simulink model "classifyRealtimeSignals"  (R2019a)
settings: Solver=VariableStepAuto  StartTime=0.0  StopTime=inf  RelTol=1e-3
undefined symbols (not defined in the file or in its folder): daq
libraries: dspfdesign x3, dspxfrm3 x3, dspnetwork x2, daqlib x1
settings Model: Creator=Kusunoki  LastModifiedBy=Owner

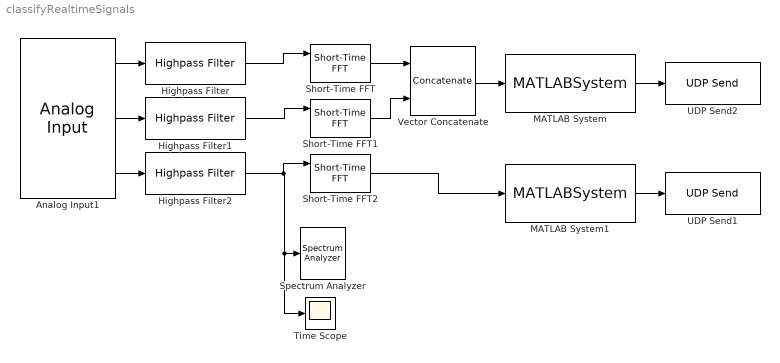
== system classifyRealtimeSignals ==
  Analog Input1 : daqlib/Analog Input  DeviceMenu=ni Dev1 (USB-6000)  Device=ni Dev1 (USB-6000)  ObjConstructor=daq.createSession('ni')  NChannelsSelected=3  Channels=1$ai0$$Dev1$1$1$1$1$#1$ai1$$Dev1$1$1$1$1$#1$ai2$$Dev1$1$1$1$1$#0$ai3$$Dev1$1$1$1$1$#0$ai4$$Dev1$1$1$1$1$#0$ai5$$Dev1$1$1$1$1$#0$ai6$$Dev1$1$1$1$1$#0$ai7$$Dev1$1$1$1$1$#  NPorts=1 per channel  SampleRate=2000  ActualRate=2000.5001  ScansPerTrigger=200  OutputTimestamp=off  AcqMode=0  NumFrameBuffer=100  OutputTriggertime=off
      settings: SourceProductName=Data Acquisition Toolbox  SourceProductBaseCode=DA
  Highpass Filter : dspfdesign/Highpass Filter  FilterType=FIR  DesignForMinimumOrder=on  FilterOrder=50  StopbandFrequency=8e3  PassbandFrequency=12e3  StopbandAttenuation=80  PassbandRipple=0.1  InheritSampleRate=off  SampleRate=44100  SimulateUsing=Interpreted execution  roundingMode=Floor  coeffsDataTypeStr=fixdt(1,16)
      settings: SourceProductName=DSP System Toolbox
  Highpass Filter1 : dspfdesign/Highpass Filter  FilterType=FIR  DesignForMinimumOrder=on  FilterOrder=50  StopbandFrequency=8e3  PassbandFrequency=12e3  StopbandAttenuation=80  PassbandRipple=0.1  InheritSampleRate=off  SampleRate=44100  SimulateUsing=Interpreted execution  roundingMode=Floor  coeffsDataTypeStr=fixdt(1,16)
      settings: SourceProductName=DSP System Toolbox
  Highpass Filter2 : dspfdesign/Highpass Filter  FilterType=FIR  DesignForMinimumOrder=on  FilterOrder=50  StopbandFrequency=8e3  PassbandFrequency=12e3  StopbandAttenuation=80  PassbandRipple=0.1  InheritSampleRate=off  SampleRate=44100  SimulateUsing=Interpreted execution  roundingMode=Floor  coeffsDataTypeStr=fixdt(1,16)
      settings: SourceProductName=DSP System Toolbox
  MATLAB System : MATLABSystem  System=NetEEG  net=[]  SimulateUsing=Code generation
      mask Type: NetEEG
      mask Display:
      | disp('NetEEG');
      | port_label('input',1,'u');
      | port_label('output',1,'y');
  MATLAB System1 : MATLABSystem  System=NetEMG  net=[]  SimulateUsing=Code generation
      mask Type: NetEMG
      mask Display:
      | disp('NetEMG');
      | port_label('input',1,'u');
      | port_label('output',1,'y');
  Short-Time FFT : dspxfrm3/Short-Time FFT  W=512  OvLap=384  M=1024
      settings: SourceProductName=DSP System Toolbox  SourceProductBaseCode=DS
  Short-Time FFT1 : dspxfrm3/Short-Time FFT  W=512  OvLap=384  M=1024
      settings: SourceProductName=DSP System Toolbox  SourceProductBaseCode=DS
  Short-Time FFT2 : dspxfrm3/Short-Time FFT  W=512  OvLap=384  M=1024
      settings: SourceProductName=DSP System Toolbox  SourceProductBaseCode=DS
  Spectrum Analyzer : SpectrumAnalyzer
  Time Scope : Scope
  UDP Send1 : dspnetwork/UDP Send  remoteURL='127.0.0.1'  remotePort=25000  localURL='0.0.0.0'  localPortSource=Automatically determine  localPort=-1  sampletime=-1  blockPlatform=[]  separateLengthPort=0
      settings: SourceProductName=Simulink
  UDP Send2 : dspnetwork/UDP Send  remoteURL='127.0.0.1'  remotePort=25000  localURL='0.0.0.0'  localPortSource=Automatically determine  localPort=-1  sampletime=-1  blockPlatform=[]  separateLengthPort=0
      settings: SourceProductName=Simulink
  Vector Concatenate : Concatenate  Mode=Multidimensional array  ConcatenateDimension=2
  wires:
  Analog Input1/1 -> Highpass Filter/1
  Highpass Filter/1 -> Short-Time FFT/1
  Highpass Filter1/1 -> Short-Time FFT1/1
  Analog Input1/2 -> Highpass Filter1/1
  Analog Input1/3 -> Highpass Filter2/1
  Short-Time FFT/1 -> Vector Concatenate/1
  Short-Time FFT1/1 -> Vector Concatenate/2
  Vector Concatenate/1 -> MATLAB System/1
  MATLAB System1/1 -> UDP Send1/1
  MATLAB System/1 -> UDP Send2/1
  Highpass Filter2/1 -> Spectrum Analyzer/1, Time Scope/1, Short-Time FFT2/1
  Short-Time FFT2/1 -> MATLAB System1/1
